simulink library "Brown_Flight_Controls_lib"  (R2025b)
settings: Solver=VariableStepAuto  StartTime=0.0  StopTime=10.0  RelTol=1e-3
undefined symbols (not defined in the file): CG, dot_sat_high, dot_sat_low, init, m, NoiseOn, prop, sat_high, sat_low, tau
libraries: $bdroot x7, matrix_library x3, simulink_extras x2, aerolibutil x1
settings Model: Creator=xzach  LastModifiedBy=zbrown

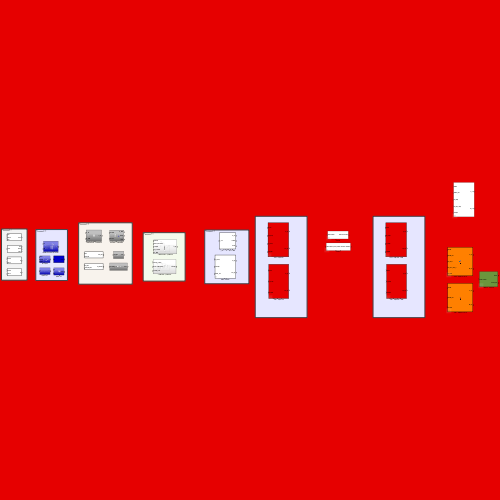
[thumbnail: Simulink's stored preview of the top-level diagram]
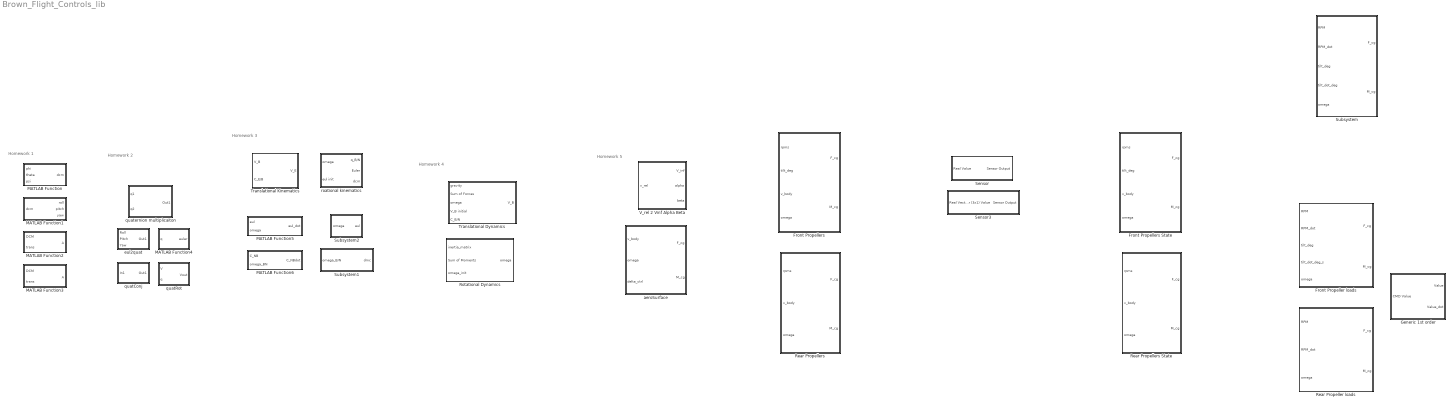
== system Brown_Flight_Controls_lib ==
  note: Homework 5
  note: Homework 4
  note: Homework 3
  note: Homework 2
  note: Homework 1
  Front Propeller loads : MATLAB Function  TreatAsAtomicUnit=on  mask{pivot_pos=prop.posFR, hub_offset=prop.hub_offset, spin_dir=prop.Rspin_dir, kT=prop.k_Thrust, kQ=prop.k_Torque, Jr=prop.Jrotor, CG=CG}
      mask prompts: pivot_pos "Pivot Position"; hub_offset "Hub offset"; spin_dir "Spin Direction"; kT "Thrust Coefficient"; kQ "reaction torque coeffecient"; Jr "rotor rotational inertia for one rotor (scalar?)"; CG "Center of Gravity"
  Front Propellers : MATLAB Function  TreatAsAtomicUnit=on  mask{pivot_pos=0, hub_offset=0, kT=0, kQ=0, CG=0, spin_dir=0}
      mask prompts: pivot_pos "Pivot position (3x3 matrix)"; hub_offset "Hub Offset length"; kT "Thrust Coefficient"; kQ "Torque Coefficient"; CG "Center of Gravity (3x1)"; spin_dir "Spin Direction of proppellers"
  Front Propellers State : MATLAB Function  TreatAsAtomicUnit=on  mask{pivot_pos=0, hub_offset=0, kT=0, kQ=0, CG=0, spin_dir=0}
      mask prompts: pivot_pos "Pivot position (3x3 matrix)"; hub_offset "Hub Offset length"; kT "Thrust Coefficient"; kQ "Torque Coefficient"; CG "Center of Gravity (3x1)"; spin_dir "Spin Direction of proppellers"
  Generic 1st order : Subsystem  mask{sat=sat_high, sat_copy=sat_low, dot_sat_high=dot_sat_high, dot_sat_low=dot_sat_low, init=init, tau=tau}
      mask prompts: sat "saturation high"; sat_copy "saturation low"; dot_sat_high "dot saturation  high"; dot_sat_low "dot saturation low"; init "initial state"; tau "time constant"
  MATLAB Function : MATLAB Function  TreatAsAtomicUnit=on
  MATLAB Function1 : MATLAB Function  TreatAsAtomicUnit=on
  MATLAB Function2 : MATLAB Function  TreatAsAtomicUnit=on
  MATLAB Function3 : MATLAB Function  TreatAsAtomicUnit=on
  MATLAB Function4 : MATLAB Function  TreatAsAtomicUnit=on
  MATLAB Function5 : MATLAB Function  TreatAsAtomicUnit=on
  MATLAB Function6 : MATLAB Function  TreatAsAtomicUnit=on
  Rear Propeller loads : MATLAB Function  TreatAsAtomicUnit=on  mask{prop_pos=prop.posRL, spin_dir=prop.Lspin_dir, kT=prop.k_Thrust, kQ=prop.k_Torque, Jr=prop.Jrotor, CG=CG}
      mask prompts: prop_pos "Propeller position"; spin_dir "Spin Direction"; kT "Thrust Coefficient"; kQ "reaction torque coeffecient"; Jr "rotor rotational inertia for one rotor (scalar?)"; CG "Center of Gravity"
  Rear Propellers : MATLAB Function  TreatAsAtomicUnit=on  mask{prop_pos=0, kT=0, kQ=0, CG=0, spin_dir=0}
      mask prompts: prop_pos "Propeller Position (3x3 matrix)"; kT "Thrust Coefficient"; kQ "Torque Coefficient"; CG "Center of Gravity 93x1)"; spin_dir "Spin Direction of proppellers"
  Rear Propellers State : MATLAB Function  TreatAsAtomicUnit=on  mask{prop_pos=0, kT=0, kQ=0, CG=0, spin_dir=0}
      mask prompts: prop_pos "Propeller Position (3x3 matrix)"; kT "Thrust Coefficient"; kQ "Torque Coefficient"; CG "Center of Gravity 93x1)"; spin_dir "Spin Direction of proppellers"
  Rotational Dynamics : Subsystem
  Sensor : Subsystem  mask{sigma=0, Ts=0, bias=0}
      mask prompts: sigma "Noise Sigma"; Ts "Sample Time"; bias "Sensor Bias"
  Sensor3 : Subsystem  mask{sigma=0, bias3=0, Ts=0}
      mask prompts: sigma "Noise Sigma"; bias3 "Sensor Bias (3x1) vec"; Ts "Sample Time"
  Subsystem : Subsystem  mask{pivot_pos=0, hub_offset=0, kT=0, kQ=0, CG=0, spin_dir=0, J_prop=0}
      mask prompts: pivot_pos "Pivot position (3x3 matrix)"; hub_offset "Hub Offset length"; kT "Thrust Coefficient"; kQ "Torque Coefficient"; CG "Center of Gravity (3x1)"; spin_dir "Spin Direction of proppellers"; J_prop "Propeller Moment of Inertia"
  Subsystem1 : Subsystem
  Subsystem2 : Subsystem
  Translational Dynamics : Subsystem
  Translational Kinematics : Subsystem
  V_rel 2 Vinf Alpha Beta : MATLAB Function  TreatAsAtomicUnit=on
  aeroSurface : MATLAB Function  TreatAsAtomicUnit=on  mask{surf=0, CG=0}
      mask prompts: surf "Surface Struct"; CG "Center of Gravity"
  eul2quat : Subsystem
  quatConj : Subsystem
  quatRot : Subsystem
  quaternion multiplicaiton : Subsystem
  roational kinematics : Subsystem

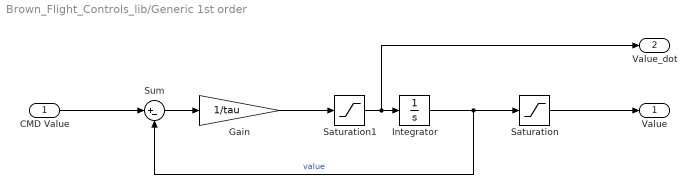
== system Brown_Flight_Controls_lib/Generic 1st order ==
  CMD Value : Inport
  Gain : Gain  Gain=1/tau
  Integrator : Integrator  InitialCondition=init
  Saturation : Saturate  UpperLimit=sat_high  LowerLimit=sat_low
  Saturation1 : Saturate  UpperLimit=dot_sat_high  LowerLimit=dot_sat_low
  Sum : Sum  Inputs=|+-
  Value : Outport
  Value_dot : Outport  Port=2
  wires:
  CMD Value/1 -> Sum/1
  Integrator/1 -> Sum/2, Saturation/1  "value"
  Sum/1 -> Gain/1
  Gain/1 -> Saturation1/1
  Saturation1/1 -> Value_dot/1, Integrator/1
  Saturation/1 -> Value/1

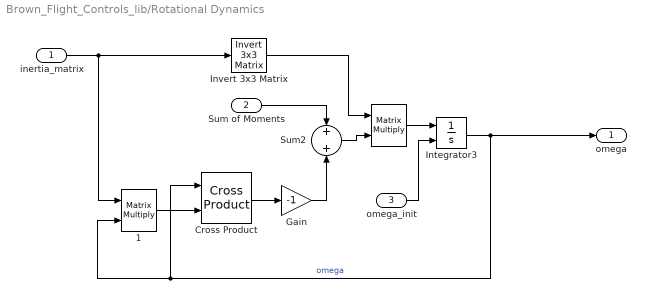
== system Brown_Flight_Controls_lib/Rotational Dynamics ==
  inertia_matrix : Inport
  Sum of Moments : Inport  Port=2
  omega_init : Inport  Port=3
  " " : Product  Multiplication=Matrix(*)
  " 1" : Product  Multiplication=Matrix(*)
  Cross Product : matrix_library/Cross Product
  Gain : Gain  Gain=-1
  Integrator3 : Integrator  InitialConditionSource=external
  Invert 3x3 Matrix : aerolibutil/Invert  3x3 Matrix
  Sum2 : Sum
  omega : Outport
  wires:
  Gain/1 -> Sum2/2
  Integrator3/1 -> omega/1, Cross Product/1, " 1"/2  "omega"
  omega_init/1 -> Integrator3/2
  Cross Product/1 -> Gain/1
  Sum of Moments/1 -> Sum2/1
  " "/1 -> Integrator3/1
  Sum2/1 -> " "/2
  inertia_matrix/1 -> Invert 3x3 Matrix/1, " 1"/1
  " 1"/1 -> Cross Product/2
  Invert 3x3 Matrix/1 -> " "/1

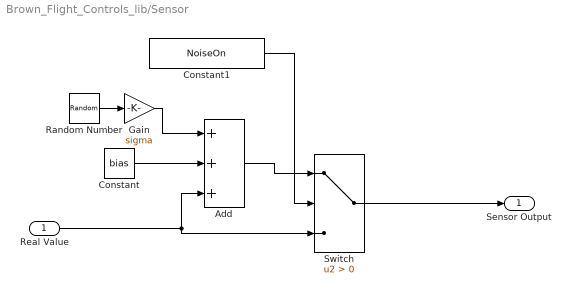
== system Brown_Flight_Controls_lib/Sensor ==
  Real Value : Inport
  Add : Sum  Inputs=+++
  Constant : Constant  Value=bias
  Constant1 : Constant  Value=NoiseOn
  Gain : Gain  Gain=sigma
  Random Number : RandomNumber  SampleTime=Ts
  Switch : Switch  Criteria=u2 > Threshold  SaturateOnIntegerOverflow=off  InputSameDT=off
  Sensor Output : Outport
  wires:
  Switch/1 -> Sensor Output/1
  Real Value/1 -> Switch/3, Add/3
  Add/1 -> Switch/1
  Constant/1 -> Add/2
  Random Number/1 -> Gain/1
  Gain/1 -> Add/1
  Constant1/1 -> Switch/2

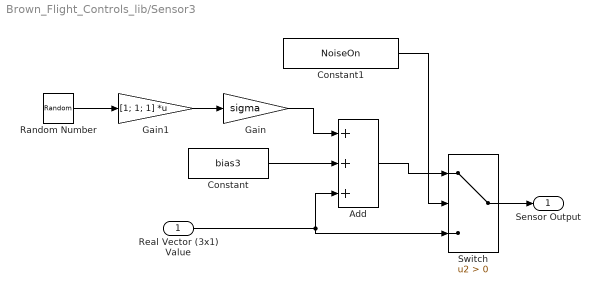
== system Brown_Flight_Controls_lib/Sensor3 ==
  Real Vector (3x1) Value : Inport
  Add : Sum  Inputs=+++
  Constant : Constant  Value=bias3
  Constant1 : Constant  Value=NoiseOn
  Gain : Gain  Gain=sigma
  Gain1 : Gain  Gain=[1; 1; 1]  Multiplication=Matrix(K*u)
  Random Number : RandomNumber  SampleTime=Ts
  Switch : Switch  Criteria=u2 > Threshold  SaturateOnIntegerOverflow=off  InputSameDT=off
  Sensor Output : Outport
  wires:
  Switch/1 -> Sensor Output/1
  Real Vector (3x1) Value/1 -> Switch/3, Add/3
  Add/1 -> Switch/1
  Constant/1 -> Add/2
  Random Number/1 -> Gain1/1
  Gain/1 -> Add/1
  Constant1/1 -> Switch/2
  Gain1/1 -> Gain/1

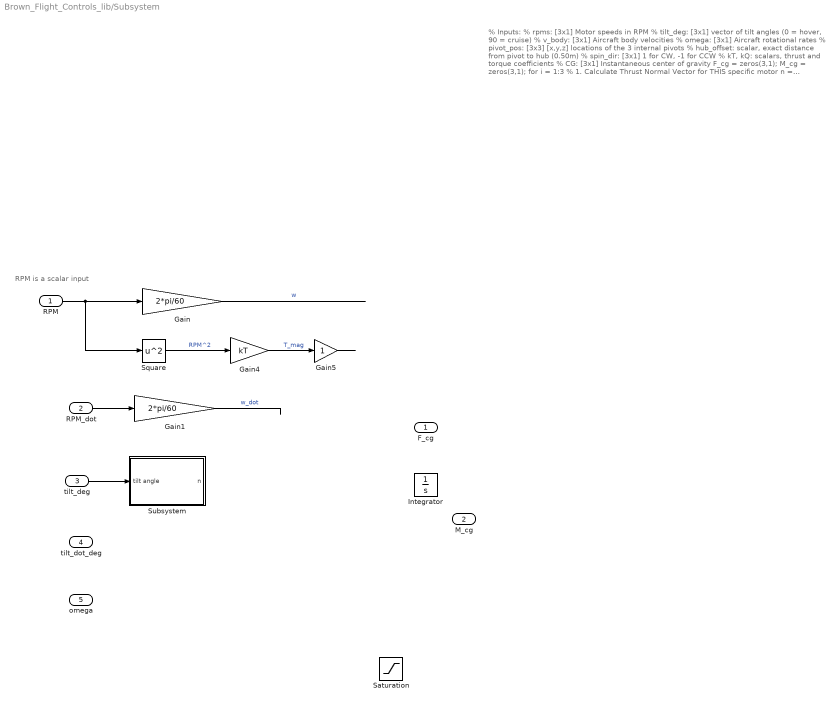
== system Brown_Flight_Controls_lib/Subsystem ==
  note: % Inputs:
      | % rpms: [3x1] Motor speeds in RPM
      | % tilt_deg: [3x1] vector of tilt angles (0 = hover, 90 = cruise)
      | % v_body: [3x1] Aircraft body velocities
      | % omega: [3x1] Aircraft rotational rates
      | % pivot_pos: [3x3] [x,y,z] locations of the 3 internal pivots
      | % hub_offset: scalar, exact distance from pivot to hub (0.50m)
      | % spin_dir: [3x1] 1 for CW, -1 for CCW
      | % kT, kQ: scalars, thrust and torque coefficients
      | % CG: [3x1] Instantaneous center of gravity
      |
      | F_cg = zeros(3,1);
      | M_cg = zeros(3,1);
      |
      | for i = 1:3
      | % 1. Calculate Thrust Normal Vector for THIS specific motor
      | n = [sind(tilt_deg(i)); 0; -cosd(tilt_deg(i))];
      |
      | % 2. Calculate Propeller Hub Location mathematically
      | % Hub pushes out from the internal pivot along the normal vector
      | r_hub = pivot_pos(i, :)' + (hub_offset * n);
      |
      | % Moment arm from CG to Hub
      | r_arm = r_hub - CG;
      |
      | % 3. Calculate Thrust/Torque
      | w = rpms(i);
      | T_mag = kT * w^2;
      | Q_mag = kQ * w^2 * spin_dir(i);
      |
      | % 4. Apply vector directions
      | F_motor = T_mag * n;
      | M_motor = -Q_mag * n; % Torque opposes spin
      |
      | % 5. Sum Forces and Moments at CG
      | F_cg = F_cg + F_motor;
      | M_cg = M_cg + cross(r_arm, F_motor) + M_motor;
      | end
      | end
  note: RPM is a scalar input
  RPM : Inport
  RPM_dot : Inport  Port=2
  tilt_deg : Inport  Port=3
  tilt_dot_deg : Inport  Port=4
  omega : Inport  Port=5
  Gain : Gain  Gain=2*pi/60
  Gain1 : Gain  Gain=2*pi/60
  Gain4 : Gain  Gain=kT
  Gain5 : Gain
  Integrator : Integrator
  Saturation : Saturate
  Square : Math  Operator=square
  Subsystem : Subsystem
  F_cg : Outport
  M_cg : Outport  Port=2
  wires:
  ? -> Integrator/1  "dRPM/dt"
  Square/1 -> Gain4/1  "RPM^2"
  RPM/1 -> Square/1, Gain/1
  Gain/1 -> ?  "w"
  RPM_dot/1 -> Gain1/1
  Gain1/1 -> ?  "w_dot"
  Gain4/1 -> Gain5/1  "T_mag"
  Gain5/1 -> ?
  tilt_deg/1 -> Subsystem/1(tilt angle)

== system Brown_Flight_Controls_lib/Subsystem1 ==
  omega_B/N : Inport
  Integrator : Integrator
  MATLAB Function6 : MATLAB Function  TreatAsAtomicUnit=on
  dmc : Outport
  wires:
  MATLAB Function6/1(C_NBdot) -> Integrator/1
  omega_B/N/1 -> MATLAB Function6/1(C_NB)
  Integrator/1 -> MATLAB Function6/2(omega_BN), dmc/1

== system Brown_Flight_Controls_lib/Subsystem2 ==
  omega : Inport
  Integrator : Integrator
  MATLAB Function5 : MATLAB Function  TreatAsAtomicUnit=on
  eul : Outport
  wires:
  MATLAB Function5/1(eul_dot) -> Integrator/1
  Integrator/1 -> eul/1, MATLAB Function5/1(eul)
  omega/1 -> MATLAB Function5/2(omega)

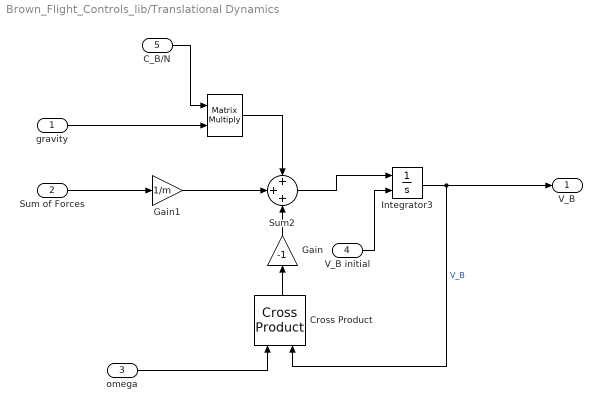
== system Brown_Flight_Controls_lib/Translational Dynamics ==
  gravity : Inport
  Sum of Forces : Inport  Port=2
  omega : Inport  Port=3
  V_B initial : Inport  Port=4
  C_B/N : Inport  Port=5
  " " : Product  Multiplication=Matrix(*)
  Cross Product : matrix_library/Cross Product
  Gain : Gain  Gain=-1
  Gain1 : Gain  Gain=1/m
  Integrator3 : Integrator  InitialConditionSource=external
  Sum2 : Sum  Inputs=+++
  V_B : Outport
  wires:
  Sum of Forces/1 -> Gain1/1
  Sum2/1 -> Integrator3/1
  Cross Product/1 -> Gain/1
  omega/1 -> Cross Product/1
  V_B initial/1 -> Integrator3/2
  Integrator3/1 -> Cross Product/2, V_B/1  "V_B"
  gravity/1 -> " "/2
  Gain/1 -> Sum2/3
  Gain1/1 -> Sum2/2
  " "/1 -> Sum2/1
  C_B/N/1 -> " "/1

== system Brown_Flight_Controls_lib/Translational Kinematics ==
  V_B : Inport
  C_E/B : Inport  Port=2
  MatrixMultiply : Product  Multiplication=Matrix(*)
  V_E : Outport
  wires:
  C_E/B/1 -> MatrixMultiply/1
  V_B/1 -> MatrixMultiply/2
  MatrixMultiply/1 -> V_E/1

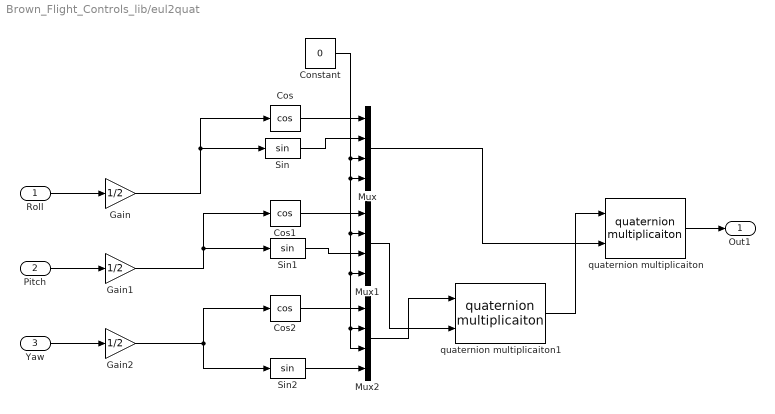
== system Brown_Flight_Controls_lib/eul2quat ==
  Roll : Inport
  Pitch : Inport  Port=2
  Yaw : Inport  Port=3
  Constant : Constant  Value=0
  Cos : Trigonometry  Operator=cos
  Cos1 : Trigonometry  Operator=cos
  Cos2 : Trigonometry  Operator=cos
  Gain : Gain  Gain=1/2
  Gain1 : Gain  Gain=1/2
  Gain2 : Gain  Gain=1/2
  Mux : Mux
  Mux1 : Mux
  Mux2 : Mux
  Sin : Trigonometry
  Sin1 : Trigonometry
  Sin2 : Trigonometry
  quaternion multiplicaiton : $bdroot/quaternion multiplicaiton  SystemSampleTime=-1  VariantActivationTime=update diagram  EmptyChoice=off  PassThrough=off  PassThroughVariantControl=(default)  EmptyChoiceVariantControl=(default)  AllowFlexibleInterface=on  Latency=0  AutoFrameSizeCalculation=off
  quaternion multiplicaiton1 : $bdroot/quaternion multiplicaiton  SystemSampleTime=-1  VariantActivationTime=update diagram  EmptyChoice=off  PassThrough=off  PassThroughVariantControl=(default)  EmptyChoiceVariantControl=(default)  AllowFlexibleInterface=on  Latency=0  AutoFrameSizeCalculation=off
  Out1 : Outport
  wires:
  Roll/1 -> Gain/1
  Pitch/1 -> Gain1/1
  Yaw/1 -> Gain2/1
  Cos/1 -> Mux/1
  Cos1/1 -> Mux1/1
  Cos2/1 -> Mux2/1
  Constant/1 -> Mux/3, Mux/4, Mux1/2, Mux2/2, Mux2/3, Mux1/4
  Gain/1 -> Sin/1, Cos/1
  Gain1/1 -> Cos1/1, Sin1/1
  Gain2/1 -> Cos2/1, Sin2/1
  Sin1/1 -> Mux1/3
  Sin/1 -> Mux/2
  Sin2/1 -> Mux2/4
  quaternion multiplicaiton/1 -> Out1/1
  Mux2/1 -> quaternion multiplicaiton1/1
  Mux1/1 -> quaternion multiplicaiton1/2
  quaternion multiplicaiton1/1 -> quaternion multiplicaiton/1
  Mux/1 -> quaternion multiplicaiton/2

== system Brown_Flight_Controls_lib/quatConj ==
  In1 : Inport
  Demux : Demux
  Gain : Gain  Gain=-1
  Mux : Mux  Inputs=3
  Mux1 : Mux  Inputs=2
  Out1 : Outport
  wires:
  Demux/3 -> Mux/2
  In1/1 -> Demux/1
  Demux/2 -> Mux/1
  Demux/4 -> Mux/3
  Demux/1 -> Mux1/1  "qw"
  Mux/1 -> Gain/1
  Mux1/1 -> Out1/1
  Gain/1 -> Mux1/2

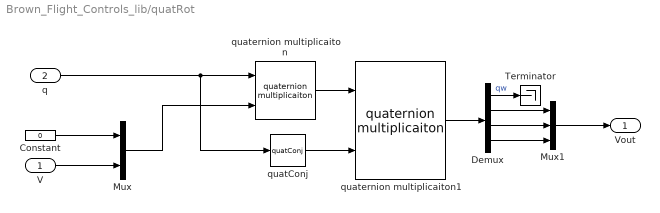
== system Brown_Flight_Controls_lib/quatRot ==
  V : Inport
  q : Inport  Port=2
  Constant : Constant  Value=0
  Demux : Demux
  Mux : Mux  Inputs=2
  Mux1 : Mux  Inputs=3
  Terminator : Terminator
  quatConj : $bdroot/quatConj  SystemSampleTime=-1  VariantActivationTime=update diagram  EmptyChoice=off  PassThrough=off  PassThroughVariantControl=(default)  EmptyChoiceVariantControl=(default)  AllowFlexibleInterface=on  Latency=0  AutoFrameSizeCalculation=off
  quaternion multiplicaiton : $bdroot/quaternion multiplicaiton  SystemSampleTime=-1  VariantActivationTime=update diagram  EmptyChoice=off  PassThrough=off  PassThroughVariantControl=(default)  EmptyChoiceVariantControl=(default)  AllowFlexibleInterface=on  Latency=0  AutoFrameSizeCalculation=off
  quaternion multiplicaiton1 : $bdroot/quaternion multiplicaiton  SystemSampleTime=-1  VariantActivationTime=update diagram  EmptyChoice=off  PassThrough=off  PassThroughVariantControl=(default)  EmptyChoiceVariantControl=(default)  AllowFlexibleInterface=on  Latency=0  AutoFrameSizeCalculation=off
  Vout : Outport
  wires:
  Constant/1 -> Mux/1
  V/1 -> Mux/2
  Mux/1 -> quaternion multiplicaiton/2
  q/1 -> quatConj/1, quaternion multiplicaiton/1
  Demux/3 -> Mux1/2
  quaternion multiplicaiton1/1 -> Demux/1
  Demux/2 -> Mux1/1
  Demux/4 -> Mux1/3
  Mux1/1 -> Vout/1
  Demux/1 -> Terminator/1  "qw"
  quaternion multiplicaiton/1 -> quaternion multiplicaiton1/1
  quatConj/1 -> quaternion multiplicaiton1/2

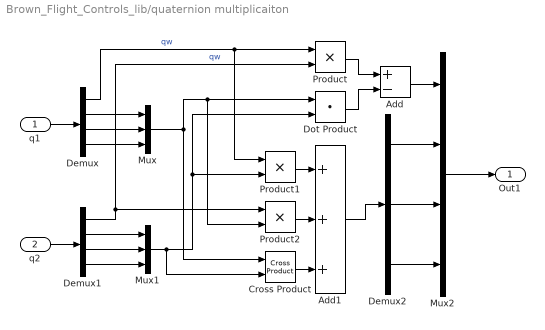
== system Brown_Flight_Controls_lib/quaternion multiplicaiton ==
  q1 : Inport
  q2 : Inport  Port=2
  Add : Sum  Inputs=+-
  Add1 : Sum  Inputs=+++
  Cross Product : matrix_library/Cross Product
  Demux : Demux
  Demux1 : Demux
  Demux2 : Demux  Outputs=3
  Dot Product : DotProduct  OutDataTypeStr=Inherit: Inherit via internal rule
  Mux : Mux  Inputs=3
  Mux1 : Mux  Inputs=3
  Mux2 : Mux
  Product : Product
  Product1 : Product
  Product2 : Product
  Out1 : Outport
  wires:
  q1/1 -> Demux/1
  Demux/1 -> Product1/1, Product/1  "qw"
  Demux/2 -> Mux/1
  Demux/3 -> Mux/2
  Demux/4 -> Mux/3
  Demux1/3 -> Mux1/2
  Demux1/2 -> Mux1/1
  Demux1/4 -> Mux1/3
  Demux1/1 -> Product2/1, Product/2  "qw"
  q2/1 -> Demux1/1
  Mux2/1 -> Out1/1
  Add/1 -> Mux2/1
  Dot Product/1 -> Add/2
  Product/1 -> Add/1
  Mux/1 -> Cross Product/1, Product2/2, Dot Product/1
  Mux1/1 -> Cross Product/2, Product1/2, Dot Product/2
  Demux2/3 -> Mux2/4
  Demux2/2 -> Mux2/3
  Demux2/1 -> Mux2/2
  Add1/1 -> Demux2/1
  Product1/1 -> Add1/1
  Product2/1 -> Add1/2
  Cross Product/1 -> Add1/3

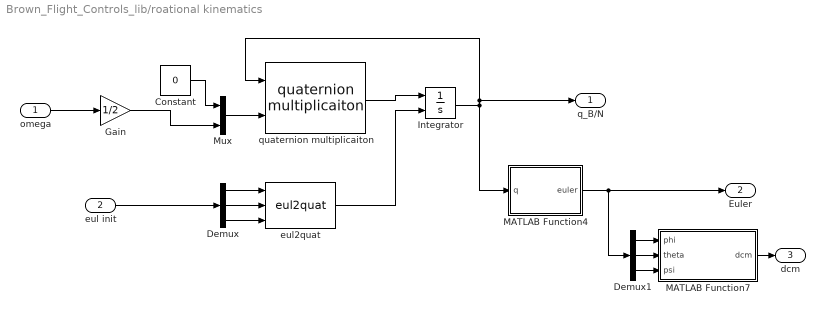
== system Brown_Flight_Controls_lib/roational kinematics ==
  omega : Inport
  eul init : Inport  Port=2
  Constant : Constant  Value=0
  Demux : Demux  Outputs=3
  Demux1 : Demux  Outputs=3
  Gain : Gain  Gain=1/2
  Integrator : Integrator  InitialConditionSource=external
  MATLAB Function4 : MATLAB Function  TreatAsAtomicUnit=on
  MATLAB Function7 : MATLAB Function  TreatAsAtomicUnit=on
  Mux : Mux  Inputs=2
  eul2quat : $bdroot/eul2quat  SystemSampleTime=-1  VariantActivationTime=update diagram  EmptyChoice=off  PassThrough=off  PassThroughVariantControl=(default)  EmptyChoiceVariantControl=(default)  AllowFlexibleInterface=on  Latency=0  AutoFrameSizeCalculation=off
  quaternion multiplicaiton : $bdroot/quaternion multiplicaiton  SystemSampleTime=-1  VariantActivationTime=update diagram  EmptyChoice=off  PassThrough=off  PassThroughVariantControl=(default)  EmptyChoiceVariantControl=(default)  AllowFlexibleInterface=on  Latency=0  AutoFrameSizeCalculation=off
  q_B/N : Outport
  Euler : Outport  Port=2
  dcm : Outport  Port=3
  wires:
  quaternion multiplicaiton/1 -> Integrator/1
  Integrator/1 -> q_B/N/1, quaternion multiplicaiton/1, MATLAB Function4/1(q)
  MATLAB Function4/1(euler) -> Demux1/1, Euler/1
  Mux/1 -> quaternion multiplicaiton/2
  Gain/1 -> Mux/2
  Constant/1 -> Mux/1
  omega/1 -> Gain/1
  eul2quat/1 -> Integrator/2
  Demux/2 -> eul2quat/2
  Demux/1 -> eul2quat/1
  Demux/3 -> eul2quat/3
  eul init/1 -> Demux/1
  Demux1/1 -> MATLAB Function7/1(phi)
  Demux1/2 -> MATLAB Function7/2(theta)
  Demux1/3 -> MATLAB Function7/3(psi)
  MATLAB Function7/1(dcm) -> dcm/1

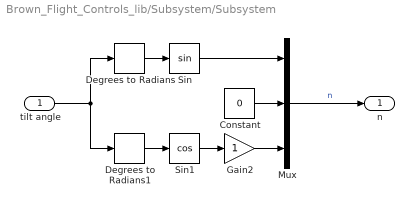
== system Brown_Flight_Controls_lib/Subsystem/Subsystem ==
  tilt angle : Inport
  Constant : Constant  Value=0
  Degrees to Radians : simulink_extras/Transformations/Degrees to Radians
  Degrees to Radians1 : simulink_extras/Transformations/Degrees to Radians
  Gain2 : Gain
  Mux : Mux  Inputs=3
  Sin : Trigonometry
  Sin1 : Trigonometry  Operator=cos
  n : Outport
  wires:
  Constant/1 -> Mux/2
  Sin1/1 -> Gain2/1
  Degrees to Radians/1 -> Sin/1
  Gain2/1 -> Mux/3
  Mux/1 -> n/1  "n"
  Sin/1 -> Mux/1
  Degrees to Radians1/1 -> Sin1/1
  tilt angle/1 -> Degrees to Radians/1, Degrees to Radians1/1

== matlab function Brown_Flight_Controls_lib/roational kinematics/MATLAB Function7 ==
  data: phi input; theta input; dcm output; psi input
function dcm  = eul2dcm(phi, theta, psi)


% Use order: ZYX
% Angles in radians
% These are rotations mapping corrdinates to World from Body frame
% Ex: Given vector V in the body frame, rotM*V is the corrdinates in the
% world frame

cy = cos(psi);  sy = sin(psi);
cp = cos(theta);sp = sin(theta);
cr = cos(phi); sr = sin(phi);

Rz = [ cy, -sy, 0;
       sy,  cy, 0;
        0,   0, 1];

Ry = [ cp, 0, sp;
        0, 1,  0;
      -sp, 0, cp];

Rx = [ 1,  0,   0;
       0, cr, -sr;
       0, sr,  cr];

dcm = Rz*Ry*Rx;

end

== matlab function Brown_Flight_Controls_lib/V_rel 2 Vinf Alpha Beta ==
  data: v_rel input; V_inf output; alpha output; beta output
function [V_inf, alpha, beta] = compute_aero_angles(v_rel)
    U_prime = v_rel(1);
    V_prime   = v_rel(2); % V' (using V_rel to avoid confusing with absolute V)
    W_prime = v_rel(3);

    V_inf = sqrt(U_prime^2 + V_prime^2 + W_prime^2);
    alpha = atan2(W_prime, U_prime);
    if V_inf > 1e-6
        beta = asin(V_prime / V_inf);
    else
        beta = 0.0;
    end
end

== matlab function Brown_Flight_Controls_lib/aeroSurface ==
  data: v_body input; omega input; delta_ctrl input; F_cg output; M_cg output; surf parameter; CG parameter
function [F_cg, M_cg] = aeroSurface(v_body, omega, delta_ctrl, surf, CG)
if nargin < 3 || isempty(delta_ctrl)
    delta_ctrl = 0;
end

if norm(v_body) < 0.1
    F_cg = [0;0;0];
    M_cg = [0;0;0];
    return;
end

ctrl_tau = 0;
CM_delta = 0;
CD_delta2 = 0;
delta_max = inf;

if isfield(surf, 'ctrl_tau') && ~isempty(surf.ctrl_tau), ctrl_tau = surf.ctrl_tau; end
if isfield(surf, 'CM_delta') && ~isempty(surf.CM_delta), CM_delta = surf.CM_delta; end
if isfield(surf, 'CD_delta2') && ~isempty(surf.CD_delta2), CD_delta2 = surf.CD_delta2; end
if isfield(surf, 'delta_max') && ~isempty(surf.delta_max), delta_max = surf.delta_max; end

delta_ctrl = min(max(delta_ctrl, -delta_max), delta_max);

r_arm = surf.pos - CG;
v_local = v_body + cross(omega, r_arm);
V2 = sum(v_local.^2);
v_mag = sqrt(V2);
v_dir = v_local / v_mag;

normal_proj = dot(v_dir, surf.n);
normal_proj = min(max(normal_proj, -1), 1);

alpha_geom = surf.i - asin(normal_proj);
alpha_eff = alpha_geom + ctrl_tau * delta_ctrl;

qS = surf.half_rho_S * V2;

CL = surf.CL0 + surf.CLa * alpha_eff;
CD = surf.CD0 + surf.CDa * (alpha_eff - surf.a0)^2 + CD_delta2 * delta_ctrl^2;
CM = surf.CM0 + surf.CMa * alpha_eff + CM_delta * delta_ctrl;

L = qS * CL;
D = qS * CD;

dir_D = -v_dir;
dir_L = surf.n - dot(surf.n, v_dir) * v_dir;
if norm(dir_L) > 0
    dir_L = dir_L / norm(dir_L);
else
    dir_L = surf.n;
end

F_surf = L * dir_L + D * dir_D;

m_axis = cross(surf.n, v_dir);
if norm(m_axis) > 0
    m_axis = m_axis / norm(m_axis);
end
M_surf = (qS * surf.c * CM) * m_axis;

F_cg = F_surf;
M_cg = M_surf + cross(r_arm, F_surf);
end

== matlab function Brown_Flight_Controls_lib/Front Propellers ==
  data: rpms input; F_cg output; tilt_deg input; v_body input; omega input; M_cg output; pivot_pos parameter; hub_offset parameter; spin_dir parameter; kT parameter; kQ parameter; CG parameter
function [F_cg, M_cg] = frontMotorGroup(rpms, tilt_deg, v_body, omega, pivot_pos, hub_offset, spin_dir, kT, kQ, CG)
    % Inputs:
    % rpms:        [3x1] Motor speeds in RPM
    % tilt_deg:    [3x1] vector of tilt angles (0 = hover, 90 = cruise)
    % v_body:      [3x1] Aircraft body velocities
    % omega:       [3x1] Aircraft rotational rates
    % pivot_pos:   [3x3] [x,y,z] locations of the 3 internal pivots 
    % hub_offset:  scalar, exact distance from pivot to hub (0.50m)
    % spin_dir:    [3x1] 1 for CW, -1 for CCW
    % kT, kQ:      scalars, thrust and torque coefficients
    % CG:          [3x1] Instantaneous center of gravity
    
    F_cg = zeros(3,1);
    M_cg = zeros(3,1);
    
    for i = 1:3
        % 1. Calculate Thrust Normal Vector for THIS specific motor
        n = [sind(tilt_deg(i)); 0; -cosd(tilt_deg(i))];
        
        % 2. Calculate Propeller Hub Location mathematically
        % Hub pushes out from the internal pivot along the normal vector
        r_hub = pivot_pos(i, :)' + (hub_offset * n);

        
        % Moment arm from CG to Hub
        r_arm = r_hub - CG;
        
        % 3. Calculate Thrust/Torque
        w = rpms(i);
        T_mag = kT * w^2;
        Q_mag = kQ * w^2 * spin_dir(i); 
        
        % 4. Apply vector directions
        F_motor = T_mag * n;
        M_motor = -Q_mag * n;  % Torque opposes spin
        
        % 5. Sum Forces and Moments at CG
        F_cg = F_cg + F_motor;
        M_cg = M_cg + cross(r_arm, F_motor) + M_motor;
    end
end

== matlab function Brown_Flight_Controls_lib/Rear Propellers ==
  data: rpms input; F_cg output; v_body input; omega input; M_cg output; spin_dir parameter; kT parameter; kQ parameter; CG parameter; prop_pos parameter
function [F_cg, M_cg] = rearMotorGroup(rpms, v_body, omega, spin_dir, kT, kQ, CG, prop_pos)
    % Inputs:
    % rpms:        [3x1] Motor speeds in RPM
    % v_body:      [3x1] Aircraft body velocities
    % omega:       [3x1] Aircraft rotational rates
    % pivot_pos:   [3x3] [x,y,z] Exact static locations of the 3 rear hubs 
    % spin_dir:    [3x1] 1 for CW, -1 for CCW
    % kT, kQ:      scalars, thrust and torque coefficients
    % CG:          [3x1] Instantaneous center of gravity
    
    F_cg = zeros(3,1);
    M_cg = zeros(3,1);
    
    % Rear motors never tilt. Thrust is permanently straight UP (-Z)
    n = [0; 0; -1];
    
    for i = 1:3
        % For the rear, pivot_pos IS the hub position (no standoff)
        r_hub = prop_pos(i, :)';
        
        % Moment arm from CG to Hub
        r_arm = r_hub - CG;
        
        % Calculate Thrust/Torque
        w = rpms(i);
        T_mag = kT * w^2;
        Q_mag = kQ * w^2 * spin_dir(i); 
        
        % Apply vector directions
        F_motor = T_mag * n;
        M_motor = -Q_mag * n;  % Torque opposes spin
        
        % Sum Forces and Moments at CG
        F_cg = F_cg + F_motor;
        M_cg = M_cg + cross(r_arm, F_motor) + M_motor;
    end
end

== matlab function Brown_Flight_Controls_lib/Front Propellers State ==
  data: rpms input; F_cg output; tilt_deg input; v_body input; omega input; M_cg output; pivot_pos parameter; hub_offset parameter; spin_dir parameter; kT parameter; kQ parameter; CG parameter
function [F_cg, M_cg] = frontMotorGroup(rpms, tilt_deg, v_body, omega, pivot_pos, hub_offset, spin_dir, kT, kQ, CG)
    % Inputs:
    % rpms:        [3x1] Motor speeds in RPM
    % tilt_deg:    [3x1] vector of tilt angles (0 = hover, 90 = cruise)
    % v_body:      [3x1] Aircraft body velocities
    % omega:       [3x1] Aircraft rotational rates
    % pivot_pos:   [3x3] [x,y,z] locations of the 3 internal pivots 
    % hub_offset:  scalar, exact distance from pivot to hub (0.50m)
    % spin_dir:    [3x1] 1 for CW, -1 for CCW
    % kT, kQ:      scalars, thrust and torque coefficients
    % CG:          [3x1] Instantaneous center of gravity
    
    F_cg = zeros(3,1);
    M_cg = zeros(3,1);
    
    for i = 1:3
        % 1. Calculate Thrust Normal Vector for THIS specific motor
        n = [sind(tilt_deg(i)); 0; -cosd(tilt_deg(i))];
        
        % 2. Calculate Propeller Hub Location mathematically
        % Hub pushes out from the internal pivot along the normal vector
        r_hub = pivot_pos(i, :)' + (hub_offset * n);

        
        % Moment arm from CG to Hub
        r_arm = r_hub - CG;
        
        % 3. Calculate Thrust/Torque
        w = rpms(i);
        T_mag = kT * w^2;
        Q_mag = kQ * w^2 * spin_dir(i); 
        
        % 4. Apply vector directions
        F_motor = T_mag * n;
        M_motor = -Q_mag * n;  % Torque opposes spin
        
        % 5. Sum Forces and Moments at CG
        F_cg = F_cg + F_motor;
        M_cg = M_cg + cross(r_arm, F_motor) + M_motor;
    end
end

== matlab function Brown_Flight_Controls_lib/Rear Propellers State ==
  data: rpms input; F_cg output; v_body input; omega input; M_cg output; spin_dir parameter; kT parameter; kQ parameter; CG parameter; prop_pos parameter
function [F_cg, M_cg] = rearMotorGroup(rpms, v_body, omega, spin_dir, kT, kQ, CG, prop_pos)
    % Inputs:
    % rpms:        [3x1] Motor speeds in RPM
    % v_body:      [3x1] Aircraft body velocities
    % omega:       [3x1] Aircraft rotational rates
    % pivot_pos:   [3x3] [x,y,z] Exact static locations of the 3 rear hubs 
    % spin_dir:    [3x1] 1 for CW, -1 for CCW
    % kT, kQ:      scalars, thrust and torque coefficients
    % CG:          [3x1] Instantaneous center of gravity
    
    F_cg = zeros(3,1);
    M_cg = zeros(3,1);
    
    % Rear motors never tilt. Thrust is permanently straight UP (-Z)
    n = [0; 0; -1];
    
    for i = 1:3
        % For the rear, pivot_pos IS the hub position (no standoff)
        r_hub = prop_pos(i, :)';
        
        % Moment arm from CG to Hub
        r_arm = r_hub - CG;
        
        % Calculate Thrust/Torque
        w = rpms(i);
        T_mag = kT * w^2;
        Q_mag = kQ * w^2 * spin_dir(i); 
        
        % Apply vector directions
        F_motor = T_mag * n;
        M_motor = -Q_mag * n;  % Torque opposes spin
        
        % Sum Forces and Moments at CG
        F_cg = F_cg + F_motor;
        M_cg = M_cg + cross(r_arm, F_motor) + M_motor;
    end
end

== matlab function Brown_Flight_Controls_lib/Front Propeller loads ==
  data: RPM input; F_cg output; RPM_dot input; tilt_deg input; tilt_dot_deg_s input; omega input; pivot_pos parameter; hub_offset parameter; spin_dir parameter; kT parameter; kQ parameter; Jr parameter; M_cg output; CG parameter
function [F_cg, M_cg] = fcn(RPM, RPM_dot, tilt_deg, tilt_dot_deg_s, omega, pivot_pos, hub_offset, spin_dir, kT, kQ, Jr, CG) ...
%#codegen
% FRONT PROP GROUP LOADS
% Inputs
%   RPM, RPM_dot        : scalar group RPM and RPM/s
%   tilt_deg            : scalar front-group tilt angle [deg]
%   tilt_dot_deg_s      : scalar front-group tilt rate [deg/s]
%   omega               : 3x1 body rates [p;q;r] in rad/s
%   CG                  : 3x1 center of gravity in body axes
% Parameters
%   pivot_pos           : 3x3, one rotor pivot per row [x y z]
%   hub_offset          : scalar hub standoff from pivot [m]
%   spin_dir            : 3x1, +1/-1 for each rotor
%   kT, kQ              : thrust / reaction-torque coefficients (RPM based)
%   Jr                  : rotor polar inertia for ONE rotor [kg*m^2]

omega = omega(:);
CG = CG(:);
spin_dir = spin_dir(:);

F_cg = zeros(3,1);
M_cg = zeros(3,1);

tilt_rad = (pi/180) * tilt_deg;
tilt_dot_rad_s = (pi/180) * tilt_dot_deg_s;

% Shared shaft direction for all three front rotors in this group
n = [sin(tilt_rad); 0; -cos(tilt_rad)];
n_dot = tilt_dot_rad_s * [cos(tilt_rad); 0; sin(tilt_rad)];

% Shared thrust / speed terms for grouped RPM
T_mag = kT * RPM * RPM;
Q_base = kQ * RPM * RPM;
Omega = (2*pi/60) * RPM;
Omega_dot = (2*pi/60) * RPM_dot;

F_motor = T_mag * n;

for i = 1:3
    s_i = spin_dir(i);
    pivot_i = pivot_pos(i,:).';

    % Rotor hub location and moment arm
    r_hub = pivot_i + hub_offset * n;
    r_arm = r_hub - CG;

    % Existing terms
    M_arm = cross(r_arm, F_motor);
    M_reaction = -(Q_base * s_i) * n;

    % Rotor angular momentum term
    % Includes:
    %   1) spin-up / spin-down torque: Jr * Omega_dot
    %   2) shaft reorientation from tilt: Jr * Omega * n_dot
    %   3) gyroscopic coupling: omega x h
    h_i = Jr * s_i * Omega * n;
    M_momentum = -(Jr * s_i * (Omega_dot * n + Omega * n_dot) + cross(omega, h_i));

    F_cg = F_cg + F_motor;
    M_cg = M_cg + M_arm + M_reaction + M_momentum;
end
end

== matlab function Brown_Flight_Controls_lib/MATLAB Function1 ==
  data: roll output; pitch output; yaw output; dcm input
function [roll, pitch, yaw] = dcm2eul(dcm)


%returns roll pitch, and yaw in the ZYX rotation order, all angles in
%radians


roll = atan2(dcm(3,2),dcm(3,3));
pitch  = asin(-dcm(3,1));
yaw = atan2(dcm(2,1),dcm(1,1));

end

== matlab function Brown_Flight_Controls_lib/Rear Propeller loads ==
  data: RPM input; F_cg output; RPM_dot input; omega input; spin_dir parameter; kT parameter; kQ parameter; Jr parameter; M_cg output; prop_pos parameter; CG parameter
function [F_cg, M_cg] = fcn(RPM, RPM_dot, omega, spin_dir, kT, kQ, Jr, prop_pos, CG)
%#codegen
% REAR PROP GROUP LOADS
% Inputs
%   RPM, RPM_dot        : scalar group RPM and RPM/s
%   omega               : 3x1 body rates [p;q;r] in rad/s
%   CG                  : 3x1 center of gravity in body axes
% Parameters
%   prop_pos            : 3x3, one rotor hub position per row [x y z]
%   spin_dir            : 3x1, +1/-1 for each rotor
%   kT, kQ              : thrust / reaction-torque coefficients (RPM based)
%   Jr                  : rotor polar inertia for ONE rotor [kg*m^2]

omega = omega(:);
CG = CG(:);
spin_dir = spin_dir(:);

F_cg = zeros(3,1);
M_cg = zeros(3,1);

% Rear shafts are fixed vertical
n = [0; 0; -1];

T_mag = kT * RPM * RPM;
Q_base = kQ * RPM * RPM;
Omega = (2*pi/60) * RPM;
Omega_dot = (2*pi/60) * RPM_dot;

F_motor = T_mag * n;

for i = 1:3
    s_i = spin_dir(i);
    hub_i = prop_pos(i,:).';

    r_arm = hub_i - CG;

    % Existing terms
    M_arm = cross(r_arm, F_motor);
    M_reaction = -(Q_base * s_i) * n;

    % Rotor angular momentum term
    % Rear shafts do not tilt, so there is no n_dot term here
    h_i = Jr * s_i * Omega * n;
    M_momentum = -(Jr * s_i * Omega_dot * n + cross(omega, h_i));

    F_cg = F_cg + F_motor;
    M_cg = M_cg + M_arm + M_reaction + M_momentum;
end
end

== matlab function Brown_Flight_Controls_lib/MATLAB Function ==
  data: phi input; theta input; dcm output; psi input
function dcm  = eul2dcm(phi, theta, psi)


% Use order: ZYX
% Angles in radians
% These are rotations mapping corrdinates to World from Body frame
% Ex: Given vector V in the body frame, rotM*V is the corrdinates in the
% world frame

cy = cos(psi);  sy = sin(psi);
cp = cos(theta);sp = sin(theta);
cr = cos(phi); sr = sin(phi);

Rz = [ cy, -sy, 0;
       sy,  cy, 0;
        0,   0, 1];

Ry = [ cp, 0, sp;
        0, 1,  0;
      -sp, 0, cp];

Rx = [ 1,  0,   0;
       0, cr, -sr;
       0, sr,  cr];

dcm = Rz*Ry*Rx;

end

== matlab function Brown_Flight_Controls_lib/MATLAB Function2 ==
  data: DCM input; A output; trans input
function A  = affine(DCM, trans)
% Builds a 4x4 affine transform matrix
% Give R_a/b (maps coordinates from b -> A)  
% and A_a/b  (orgin of frame b  expressed in a) 
% for a tranform that works as Va = A_a/b*[Vb; 1]


A = [DCM,   trans;
     zeros(1,3), 1];
end

== matlab function Brown_Flight_Controls_lib/MATLAB Function3 ==
  data: DCM input; A output; trans input
function A  = affineInv(DCM, trans)
% Builds a 4x4 affine transform matrix
% Give R_a/b (maps coordinates from b -> A)  
% and A_a/b  (orgin of frame b  expressed in a) 
% for a tranform that works as Va = A_a/b*[Vb; 1]


A = [DCM',   -DCM'*trans;
     zeros(1,3), 1];
end

== matlab function Brown_Flight_Controls_lib/MATLAB Function4 ==
  data: q input; euler output
function euler = quat2euler(q)
    w = q(1);
    x = q(2);
    y = q(3);
    z = q(4);

    %gimbal lock calc
    sinp = 2 * (w * y - z * x);
    
    if abs(sinp) >= 1
        % Gimbal Lock 
        pitch = sign(sinp) * (pi / 2);
        roll = 0;

        yaw = 2 * atan2(x, w);
    else
        pitch = asin(sinp);

        sinr_cosp = 2 * (w * x + y * z);
        cosr_cosp = 1 - 2 * (x * x + y * y);
        roll = atan2(sinr_cosp, cosr_cosp);
        
        siny_cosp = 2 * (w * z + x * y);
        cosy_cosp = 1 - 2 * (y * y + z * z);
        yaw = atan2(siny_cosp, cosy_cosp);
    end

    euler = [roll; pitch; yaw];
end

== matlab function Brown_Flight_Controls_lib/MATLAB Function5 ==
  data: eul input; eul_dot output; omega input
function eul_dot = RK_theta_dot(eul, omega)
phi = eul(1); th = eul(2);
p = omega(1); q = omega(2); r = omega(3);

T = [ 1,  sin(phi)*tan(th),  cos(phi)*tan(th);
      0,  cos(phi),        -sin(phi);
      0,  sin(phi)/cos(th), cos(phi)/cos(th) ];

eul_dot = T*[p;q;r];
end

== matlab function Brown_Flight_Controls_lib/MATLAB Function6 ==
  data: C_NB input; C_NBdot output; omega_BN input

function C_NBdot = dcmDot(C_NB, omega_BN)
W = [ 0, -omega_BN(3),  omega_BN(2);
      omega_BN(3),  0, -omega_BN(1);
     -omega_BN(2),  omega_BN(1),  0 ];

C_NBdot = W*C_NB;
end

== matlab function Brown_Flight_Controls_lib/roational kinematics/MATLAB Function4 ==
  data: q input; euler output
function euler = quat2euler(q)
    w = q(1);
    x = q(2);
    y = q(3);
    z = q(4);

    %gimbal lock calc
    sinp = 2 * (w * y - z * x);
    
    if abs(sinp) >= 1
        % Gimbal Lock 
        pitch = sign(sinp) * (pi / 2);
        roll = 0;

        yaw = 2 * atan2(x, w);
    else
        pitch = asin(sinp);

        sinr_cosp = 2 * (w * x + y * z);
        cosr_cosp = 1 - 2 * (x * x + y * y);
        roll = atan2(sinr_cosp, cosr_cosp);
        
        siny_cosp = 2 * (w * z + x * y);
        cosy_cosp = 1 - 2 * (y * y + z * z);
        yaw = atan2(siny_cosp, cosy_cosp);
    end

    euler = [roll; pitch; yaw];
end

== matlab function Brown_Flight_Controls_lib/Subsystem1/MATLAB Function6 ==
  data: C_NB input; C_NBdot output; omega_BN input

function C_NBdot = dcmDot(C_NB, omega_BN)
W = [ 0, -omega_BN(3),  omega_BN(2);
      omega_BN(3),  0, -omega_BN(1);
     -omega_BN(2),  omega_BN(1),  0 ];

C_NBdot = W*C_NB;
end

== matlab function Brown_Flight_Controls_lib/Subsystem2/MATLAB Function5 ==
  data: eul input; eul_dot output; omega input
function eul_dot = RK_theta_dot(eul, omega)
phi = eul(1); th = eul(2);
p = omega(1); q = omega(2); r = omega(3);

T = [ 1,  sin(phi)*tan(th),  cos(phi)*tan(th);
      0,  cos(phi),        -sin(phi);
      0,  sin(phi)/cos(th), cos(phi)/cos(th) ];

eul_dot = T*[p;q;r];
end
